simulink model "ctrl_student_HIL"  (R2015a)
settings: Solver=ode3  StartTime=0.0  StopTime=inf  RelTol=1e-3
libraries: dspstat3 x1, simulink x1
(part 2 of 3)

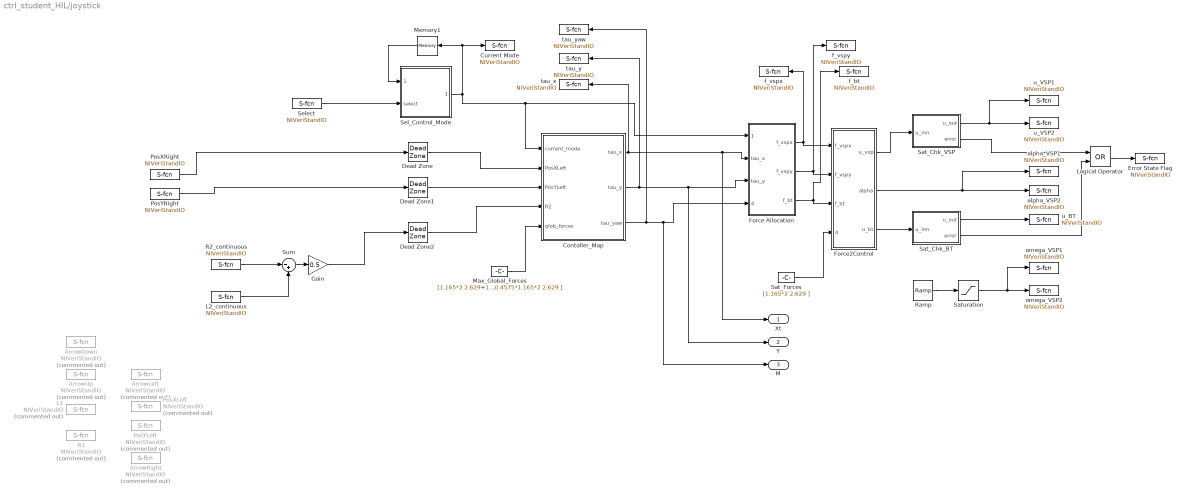
== system ctrl_student_HIL/joystick ==
  ArrowDown : S-Function  Priority=9  Commented=on  FunctionName=NIVeriStandIO  Parameters=width dtype portnum stime stype btype  mask(NI VeriStand Inport){portnum=9, width=-1, stime=-1, dtype=auto, stype=auto, btype=1}
      mask prompts: portnum "Port number:"; width "Port dimensions (-1 for dynamically sized):"; stime "Sample time (-1 for inherited):"; dtype "Data type:"; stype "Signal type:"; btype "Block type:"
      mask help: Use this inport on any level of nested subsystems to allow NI VeriStand software to map signals to it.
      mask init:
      | NIVeriStandIO_init;
      settings: CopyFcn=NIVeriStand_MDL_functions('', 'IO_copy');  DeleteFcn=NIVeriStand_MDL_functions('', 'IO_delete');  MoveFcn=set_param(gcb, 'Mask', 'on');
      mask Callback portnum: NIVeriStand_MDL_functions('', 'IO_setportnum');
      mask TypeOptions dtype: auto | double | single | int8 | uint8 | int16 | uint16 | int32 | uint32 | boolean
      mask Callback dtype: NIVeriStand_MDL_functions('', 'IO_booleansignal');
      mask TypeOptions stype: auto | real | complex
      mask Display:
      | patch([-x x], [-y y], [.90980 .81960 .32156]);
      | plot([xrad -x x xrad], [yrad -y y yrad]);
      | fprintf('NI In%d', portnum);
  ArrowLeft : S-Function  Priority=11  Commented=on  FunctionName=NIVeriStandIO  Parameters=width dtype portnum stime stype btype  mask(NI VeriStand Inport){portnum=11, width=-1, stime=-1, dtype=auto, stype=auto, btype=1}
      mask prompts: portnum "Port number:"; width "Port dimensions (-1 for dynamically sized):"; stime "Sample time (-1 for inherited):"; dtype "Data type:"; stype "Signal type:"; btype "Block type:"
      mask help: Use this inport on any level of nested subsystems to allow NI VeriStand software to map signals to it.
      mask init:
      | NIVeriStandIO_init;
      settings: CopyFcn=NIVeriStand_MDL_functions('', 'IO_copy');  DeleteFcn=NIVeriStand_MDL_functions('', 'IO_delete');  MoveFcn=set_param(gcb, 'Mask', 'on');
      mask Callback portnum: NIVeriStand_MDL_functions('', 'IO_setportnum');
      mask TypeOptions dtype: auto | double | single | int8 | uint8 | int16 | uint16 | int32 | uint32 | boolean
      mask Callback dtype: NIVeriStand_MDL_functions('', 'IO_booleansignal');
      mask TypeOptions stype: auto | real | complex
      mask Display:
      | patch([-x x], [-y y], [.90980 .81960 .32156]);
      | plot([xrad -x x xrad], [yrad -y y yrad]);
      | fprintf('NI In%d', portnum);
  ArrowRight : S-Function  Priority=12  Commented=on  FunctionName=NIVeriStandIO  Parameters=width dtype portnum stime stype btype  mask(NI VeriStand Inport){portnum=12, width=-1, stime=-1, dtype=auto, stype=auto, btype=1}
      mask prompts: portnum "Port number:"; width "Port dimensions (-1 for dynamically sized):"; stime "Sample time (-1 for inherited):"; dtype "Data type:"; stype "Signal type:"; btype "Block type:"
      mask help: Use this inport on any level of nested subsystems to allow NI VeriStand software to map signals to it.
      mask init:
      | NIVeriStandIO_init;
      settings: CopyFcn=NIVeriStand_MDL_functions('', 'IO_copy');  DeleteFcn=NIVeriStand_MDL_functions('', 'IO_delete');  MoveFcn=set_param(gcb, 'Mask', 'on');
      mask Callback portnum: NIVeriStand_MDL_functions('', 'IO_setportnum');
      mask TypeOptions dtype: auto | double | single | int8 | uint8 | int16 | uint16 | int32 | uint32 | boolean
      mask Callback dtype: NIVeriStand_MDL_functions('', 'IO_booleansignal');
      mask TypeOptions stype: auto | real | complex
      mask Display:
      | patch([-x x], [-y y], [.90980 .81960 .32156]);
      | plot([xrad -x x xrad], [yrad -y y yrad]);
      | fprintf('NI In%d', portnum);
  ArrowUp : S-Function  Priority=10  Commented=on  FunctionName=NIVeriStandIO  Parameters=width dtype portnum stime stype btype  mask(NI VeriStand Inport){portnum=10, width=-1, stime=-1, dtype=auto, stype=auto, btype=1}
      mask prompts: portnum "Port number:"; width "Port dimensions (-1 for dynamically sized):"; stime "Sample time (-1 for inherited):"; dtype "Data type:"; stype "Signal type:"; btype "Block type:"
      mask help: Use this inport on any level of nested subsystems to allow NI VeriStand software to map signals to it.
      mask init:
      | NIVeriStandIO_init;
      settings: CopyFcn=NIVeriStand_MDL_functions('', 'IO_copy');  DeleteFcn=NIVeriStand_MDL_functions('', 'IO_delete');  MoveFcn=set_param(gcb, 'Mask', 'on');
      mask Callback portnum: NIVeriStand_MDL_functions('', 'IO_setportnum');
      mask TypeOptions dtype: auto | double | single | int8 | uint8 | int16 | uint16 | int32 | uint32 | boolean
      mask Callback dtype: NIVeriStand_MDL_functions('', 'IO_booleansignal');
      mask TypeOptions stype: auto | real | complex
      mask Display:
      | patch([-x x], [-y y], [.90980 .81960 .32156]);
      | plot([xrad -x x xrad], [yrad -y y yrad]);
      | fprintf('NI In%d', portnum);
  Contoller_Map : MATLAB Function  TreatAsAtomicUnit=on
  "Current Mode " : S-Function  Priority=8  FunctionName=NIVeriStandIO  Parameters=width dtype portnum stime stype btype  mask(NI VeriStand Outport){portnum=8, width=-1, stime=-1, dtype=auto, stype=auto, btype=0}
      mask prompts: portnum "Port number:"; width "Port dimensions (-1 for dynamically sized):"; stime "Sample time (-1 for inherited):"; dtype "Data type:"; stype "Signal type:"; btype "Block type:"
      mask help: Use this outport on any level of nested subsystems to allow NI VeriStand software to map signals to it.
      mask init:
      | NIVeriStandIO_init;
      settings: CopyFcn=NIVeriStand_MDL_functions('', 'IO_copy');  DeleteFcn=NIVeriStand_MDL_functions('', 'IO_delete');  MoveFcn=set_param(gcb, 'Mask', 'on');
      mask Callback portnum: NIVeriStand_MDL_functions('', 'IO_setportnum');
      mask TypeOptions dtype: auto | double | single | int8 | uint8 | int16 | uint16 | int32 | uint32 | boolean
      mask Callback dtype: NIVeriStand_MDL_functions('', 'IO_booleansignal');
      mask TypeOptions stype: auto | real | complex
      mask Display:
      | patch([-x x], [-y y], [.90980 .81960 .32156]);
      | plot([xrad -x x xrad], [yrad -y y yrad]);
      | fprintf('NI Out%d', portnum);
  Dead Zone : DeadZone  LowerValue=-0.05  UpperValue=0.05  SaturateOnIntegerOverflow=on
  Dead Zone1 : DeadZone  LowerValue=-0.05  UpperValue=0.05  SaturateOnIntegerOverflow=on
  Dead Zone2 : DeadZone  LowerValue=-0.05  UpperValue=0.05  SaturateOnIntegerOverflow=on
  Error State Flag : S-Function  Priority=9  FunctionName=NIVeriStandIO  Parameters=width dtype portnum stime stype btype  mask(NI VeriStand Outport){portnum=9, width=-1, stime=-1, dtype=boolean, stype=auto, btype=0}
      mask prompts: portnum "Port number:"; width "Port dimensions (-1 for dynamically sized):"; stime "Sample time (-1 for inherited):"; dtype "Data type:"; stype "Signal type:"; btype "Block type:"
      mask help: Use this outport on any level of nested subsystems to allow NI VeriStand software to map signals to it.
      mask init:
      | NIVeriStandIO_init;
      settings: CopyFcn=NIVeriStand_MDL_functions('', 'IO_copy');  DeleteFcn=NIVeriStand_MDL_functions('', 'IO_delete');  MoveFcn=set_param(gcb, 'Mask', 'on');
      mask Callback portnum: NIVeriStand_MDL_functions('', 'IO_setportnum');
      mask TypeOptions dtype: auto | double | single | int8 | uint8 | int16 | uint16 | int32 | uint32 | boolean
      mask Callback dtype: NIVeriStand_MDL_functions('', 'IO_booleansignal');
      mask TypeOptions stype: auto | real | complex
      mask Display:
      | patch([-x x], [-y y], [.90980 .81960 .32156]);
      | plot([xrad -x x xrad], [yrad -y y yrad]);
      | fprintf('NI Out%d', portnum);
  Force Allocation : MATLAB Function  TreatAsAtomicUnit=on
  Force2Control : MATLAB Function  TreatAsAtomicUnit=on
  Gain : Gain  Gain=0.5
  L1 : S-Function  Priority=7  Commented=on  FunctionName=NIVeriStandIO  Parameters=width dtype portnum stime stype btype  mask(NI VeriStand Inport){portnum=7, width=-1, stime=-1, dtype=auto, stype=auto, btype=1}
      mask prompts: portnum "Port number:"; width "Port dimensions (-1 for dynamically sized):"; stime "Sample time (-1 for inherited):"; dtype "Data type:"; stype "Signal type:"; btype "Block type:"
      mask help: Use this inport on any level of nested subsystems to allow NI VeriStand software to map signals to it.
      mask init:
      | NIVeriStandIO_init;
      settings: CopyFcn=NIVeriStand_MDL_functions('', 'IO_copy');  DeleteFcn=NIVeriStand_MDL_functions('', 'IO_delete');  MoveFcn=set_param(gcb, 'Mask', 'on');
      mask Callback portnum: NIVeriStand_MDL_functions('', 'IO_setportnum');
      mask TypeOptions dtype: auto | double | single | int8 | uint8 | int16 | uint16 | int32 | uint32 | boolean
      mask Callback dtype: NIVeriStand_MDL_functions('', 'IO_booleansignal');
      mask TypeOptions stype: auto | real | complex
      mask Display:
      | patch([-x x], [-y y], [.90980 .81960 .32156]);
      | plot([xrad -x x xrad], [yrad -y y yrad]);
      | fprintf('NI In%d', portnum);
  L2_continuous : S-Function  Priority=1  FunctionName=NIVeriStandIO  Parameters=width dtype portnum stime stype btype  mask(NI VeriStand Inport){portnum=1, width=-1, stime=-1, dtype=auto, stype=auto, btype=1}
      mask prompts: portnum "Port number:"; width "Port dimensions (-1 for dynamically sized):"; stime "Sample time (-1 for inherited):"; dtype "Data type:"; stype "Signal type:"; btype "Block type:"
      mask help: Use this inport on any level of nested subsystems to allow NI VeriStand software to map signals to it.
      mask init:
      | NIVeriStandIO_init;
      settings: CopyFcn=NIVeriStand_MDL_functions('', 'IO_copy');  DeleteFcn=NIVeriStand_MDL_functions('', 'IO_delete');  MoveFcn=set_param(gcb, 'Mask', 'on');
      mask Callback portnum: NIVeriStand_MDL_functions('', 'IO_setportnum');
      mask TypeOptions dtype: auto | double | single | int8 | uint8 | int16 | uint16 | int32 | uint32 | boolean
      mask Callback dtype: NIVeriStand_MDL_functions('', 'IO_booleansignal');
      mask TypeOptions stype: auto | real | complex
      mask Display:
      | patch([-x x], [-y y], [.90980 .81960 .32156]);
      | plot([xrad -x x xrad], [yrad -y y yrad]);
      | fprintf('NI In%d', portnum);
  Logical Operator : Logic  Operator=OR  AllPortsSameDT=off  OutDataTypeStr=boolean
  Max_Global_Forces : Constant  Value=[1.165*2 2.629+1.165*2 0.3875*2.629+0.4575*1.165*2 2.629 ]
  Memory1 : Memory  X0=2
  PosXLeft : S-Function  Priority=5  Commented=on  FunctionName=NIVeriStandIO  Parameters=width dtype portnum stime stype btype  mask(NI VeriStand Inport){portnum=5, width=-1, stime=-1, dtype=auto, stype=auto, btype=1}
      mask prompts: portnum "Port number:"; width "Port dimensions (-1 for dynamically sized):"; stime "Sample time (-1 for inherited):"; dtype "Data type:"; stype "Signal type:"; btype "Block type:"
      mask help: Use this inport on any level of nested subsystems to allow NI VeriStand software to map signals to it.
      mask init:
      | NIVeriStandIO_init;
      settings: CopyFcn=NIVeriStand_MDL_functions('', 'IO_copy');  DeleteFcn=NIVeriStand_MDL_functions('', 'IO_delete');  MoveFcn=set_param(gcb, 'Mask', 'on');
      mask Callback portnum: NIVeriStand_MDL_functions('', 'IO_setportnum');
      mask TypeOptions dtype: auto | double | single | int8 | uint8 | int16 | uint16 | int32 | uint32 | boolean
      mask Callback dtype: NIVeriStand_MDL_functions('', 'IO_booleansignal');
      mask TypeOptions stype: auto | real | complex
      mask Display:
      | patch([-x x], [-y y], [.90980 .81960 .32156]);
      | plot([xrad -x x xrad], [yrad -y y yrad]);
      | fprintf('NI In%d', portnum);
  PosXRight : S-Function  Priority=2  FunctionName=NIVeriStandIO  Parameters=width dtype portnum stime stype btype  mask(NI VeriStand Inport){portnum=2, width=-1, stime=-1, dtype=auto, stype=auto, btype=1}
      mask prompts: portnum "Port number:"; width "Port dimensions (-1 for dynamically sized):"; stime "Sample time (-1 for inherited):"; dtype "Data type:"; stype "Signal type:"; btype "Block type:"
      mask help: Use this inport on any level of nested subsystems to allow NI VeriStand software to map signals to it.
      mask init:
      | NIVeriStandIO_init;
      settings: CopyFcn=NIVeriStand_MDL_functions('', 'IO_copy');  DeleteFcn=NIVeriStand_MDL_functions('', 'IO_delete');  MoveFcn=set_param(gcb, 'Mask', 'on');
      mask Callback portnum: NIVeriStand_MDL_functions('', 'IO_setportnum');
      mask TypeOptions dtype: auto | double | single | int8 | uint8 | int16 | uint16 | int32 | uint32 | boolean
      mask Callback dtype: NIVeriStand_MDL_functions('', 'IO_booleansignal');
      mask TypeOptions stype: auto | real | complex
      mask Display:
      | patch([-x x], [-y y], [.90980 .81960 .32156]);
      | plot([xrad -x x xrad], [yrad -y y yrad]);
      | fprintf('NI In%d', portnum);
  PosYLeft : S-Function  Priority=6  Commented=on  FunctionName=NIVeriStandIO  Parameters=width dtype portnum stime stype btype  mask(NI VeriStand Inport){portnum=6, width=-1, stime=-1, dtype=auto, stype=auto, btype=1}
      mask prompts: portnum "Port number:"; width "Port dimensions (-1 for dynamically sized):"; stime "Sample time (-1 for inherited):"; dtype "Data type:"; stype "Signal type:"; btype "Block type:"
      mask help: Use this inport on any level of nested subsystems to allow NI VeriStand software to map signals to it.
      mask init:
      | NIVeriStandIO_init;
      settings: CopyFcn=NIVeriStand_MDL_functions('', 'IO_copy');  DeleteFcn=NIVeriStand_MDL_functions('', 'IO_delete');  MoveFcn=set_param(gcb, 'Mask', 'on');
      mask Callback portnum: NIVeriStand_MDL_functions('', 'IO_setportnum');
      mask TypeOptions dtype: auto | double | single | int8 | uint8 | int16 | uint16 | int32 | uint32 | boolean
      mask Callback dtype: NIVeriStand_MDL_functions('', 'IO_booleansignal');
      mask TypeOptions stype: auto | real | complex
      mask Display:
      | patch([-x x], [-y y], [.90980 .81960 .32156]);
      | plot([xrad -x x xrad], [yrad -y y yrad]);
      | fprintf('NI In%d', portnum);
  PosYRight : S-Function  Priority=3  FunctionName=NIVeriStandIO  Parameters=width dtype portnum stime stype btype  mask(NI VeriStand Inport){portnum=3, width=-1, stime=-1, dtype=auto, stype=auto, btype=1}
      mask prompts: portnum "Port number:"; width "Port dimensions (-1 for dynamically sized):"; stime "Sample time (-1 for inherited):"; dtype "Data type:"; stype "Signal type:"; btype "Block type:"
      mask help: Use this inport on any level of nested subsystems to allow NI VeriStand software to map signals to it.
      mask init:
      | NIVeriStandIO_init;
      settings: CopyFcn=NIVeriStand_MDL_functions('', 'IO_copy');  DeleteFcn=NIVeriStand_MDL_functions('', 'IO_delete');  MoveFcn=set_param(gcb, 'Mask', 'on');
      mask Callback portnum: NIVeriStand_MDL_functions('', 'IO_setportnum');
      mask TypeOptions dtype: auto | double | single | int8 | uint8 | int16 | uint16 | int32 | uint32 | boolean
      mask Callback dtype: NIVeriStand_MDL_functions('', 'IO_booleansignal');
      mask TypeOptions stype: auto | real | complex
      mask Display:
      | patch([-x x], [-y y], [.90980 .81960 .32156]);
      | plot([xrad -x x xrad], [yrad -y y yrad]);
      | fprintf('NI In%d', portnum);
  R1 : S-Function  Priority=8  Commented=on  FunctionName=NIVeriStandIO  Parameters=width dtype portnum stime stype btype  mask(NI VeriStand Inport){portnum=8, width=-1, stime=-1, dtype=auto, stype=auto, btype=1}
      mask prompts: portnum "Port number:"; width "Port dimensions (-1 for dynamically sized):"; stime "Sample time (-1 for inherited):"; dtype "Data type:"; stype "Signal type:"; btype "Block type:"
      mask help: Use this inport on any level of nested subsystems to allow NI VeriStand software to map signals to it.
      mask init:
      | NIVeriStandIO_init;
      settings: CopyFcn=NIVeriStand_MDL_functions('', 'IO_copy');  DeleteFcn=NIVeriStand_MDL_functions('', 'IO_delete');  MoveFcn=set_param(gcb, 'Mask', 'on');
      mask Callback portnum: NIVeriStand_MDL_functions('', 'IO_setportnum');
      mask TypeOptions dtype: auto | double | single | int8 | uint8 | int16 | uint16 | int32 | uint32 | boolean
      mask Callback dtype: NIVeriStand_MDL_functions('', 'IO_booleansignal');
      mask TypeOptions stype: auto | real | complex
      mask Display:
      | patch([-x x], [-y y], [.90980 .81960 .32156]);
      | plot([xrad -x x xrad], [yrad -y y yrad]);
      | fprintf('NI In%d', portnum);
  R2_continuous : S-Function  Priority=4  FunctionName=NIVeriStandIO  Parameters=width dtype portnum stime stype btype  mask(NI VeriStand Inport){portnum=4, width=-1, stime=-1, dtype=auto, stype=auto, btype=1}
      mask prompts: portnum "Port number:"; width "Port dimensions (-1 for dynamically sized):"; stime "Sample time (-1 for inherited):"; dtype "Data type:"; stype "Signal type:"; btype "Block type:"
      mask help: Use this inport on any level of nested subsystems to allow NI VeriStand software to map signals to it.
      mask init:
      | NIVeriStandIO_init;
      settings: CopyFcn=NIVeriStand_MDL_functions('', 'IO_copy');  DeleteFcn=NIVeriStand_MDL_functions('', 'IO_delete');  MoveFcn=set_param(gcb, 'Mask', 'on');
      mask Callback portnum: NIVeriStand_MDL_functions('', 'IO_setportnum');
      mask TypeOptions dtype: auto | double | single | int8 | uint8 | int16 | uint16 | int32 | uint32 | boolean
      mask Callback dtype: NIVeriStand_MDL_functions('', 'IO_booleansignal');
      mask TypeOptions stype: auto | real | complex
      mask Display:
      | patch([-x x], [-y y], [.90980 .81960 .32156]);
      | plot([xrad -x x xrad], [yrad -y y yrad]);
      | fprintf('NI In%d', portnum);
  Ramp : simulink/Sources/Ramp  slope=0.1  start=0  X0=0
  Sat_Chk_BT : MATLAB Function  TreatAsAtomicUnit=on
  Sat_Chk_VSP : MATLAB Function  TreatAsAtomicUnit=on
  Sat_Forces : Constant  Value=[1.165*2 2.629 ]
  Saturation : Saturate  UpperLimit=0.3  LowerLimit=0
  Sel_Control_Mode : MATLAB Function  TreatAsAtomicUnit=on
  Select : S-Function  Priority=13  FunctionName=NIVeriStandIO  Parameters=width dtype portnum stime stype btype  mask(NI VeriStand Inport){portnum=13, width=-1, stime=-1, dtype=auto, stype=auto, btype=1}
      mask prompts: portnum "Port number:"; width "Port dimensions (-1 for dynamically sized):"; stime "Sample time (-1 for inherited):"; dtype "Data type:"; stype "Signal type:"; btype "Block type:"
      mask help: Use this inport on any level of nested subsystems to allow NI VeriStand software to map signals to it.
      mask init:
      | NIVeriStandIO_init;
      settings: CopyFcn=NIVeriStand_MDL_functions('', 'IO_copy');  DeleteFcn=NIVeriStand_MDL_functions('', 'IO_delete');  MoveFcn=set_param(gcb, 'Mask', 'on');
      mask Callback portnum: NIVeriStand_MDL_functions('', 'IO_setportnum');
      mask TypeOptions dtype: auto | double | single | int8 | uint8 | int16 | uint16 | int32 | uint32 | boolean
      mask Callback dtype: NIVeriStand_MDL_functions('', 'IO_booleansignal');
      mask TypeOptions stype: auto | real | complex
      mask Display:
      | patch([-x x], [-y y], [.90980 .81960 .32156]);
      | plot([xrad -x x xrad], [yrad -y y yrad]);
      | fprintf('NI In%d', portnum);
  Sum : Sum  Inputs=|-+
  alpha_VSP1 : S-Function  Priority=4  FunctionName=NIVeriStandIO  Parameters=width dtype portnum stime stype btype  mask(NI VeriStand Outport){portnum=4, width=-1, stime=-1, dtype=auto, stype=auto, btype=0}
      mask prompts: portnum "Port number:"; width "Port dimensions (-1 for dynamically sized):"; stime "Sample time (-1 for inherited):"; dtype "Data type:"; stype "Signal type:"; btype "Block type:"
      mask help: Use this outport on any level of nested subsystems to allow NI VeriStand software to map signals to it.
      mask init:
      | NIVeriStandIO_init;
      settings: CopyFcn=NIVeriStand_MDL_functions('', 'IO_copy');  DeleteFcn=NIVeriStand_MDL_functions('', 'IO_delete');  MoveFcn=set_param(gcb, 'Mask', 'on');
      mask Callback portnum: NIVeriStand_MDL_functions('', 'IO_setportnum');
      mask TypeOptions dtype: auto | double | single | int8 | uint8 | int16 | uint16 | int32 | uint32 | boolean
      mask Callback dtype: NIVeriStand_MDL_functions('', 'IO_booleansignal');
      mask TypeOptions stype: auto | real | complex
      mask Display:
      | patch([-x x], [-y y], [.90980 .81960 .32156]);
      | plot([xrad -x x xrad], [yrad -y y yrad]);
      | fprintf('NI Out%d', portnum);
  alpha_VSP2 : S-Function  Priority=5  FunctionName=NIVeriStandIO  Parameters=width dtype portnum stime stype btype  mask(NI VeriStand Outport){portnum=5, width=-1, stime=-1, dtype=auto, stype=auto, btype=0}
      mask prompts: portnum "Port number:"; width "Port dimensions (-1 for dynamically sized):"; stime "Sample time (-1 for inherited):"; dtype "Data type:"; stype "Signal type:"; btype "Block type:"
      mask help: Use this outport on any level of nested subsystems to allow NI VeriStand software to map signals to it.
      mask init:
      | NIVeriStandIO_init;
      settings: CopyFcn=NIVeriStand_MDL_functions('', 'IO_copy');  DeleteFcn=NIVeriStand_MDL_functions('', 'IO_delete');  MoveFcn=set_param(gcb, 'Mask', 'on');
      mask Callback portnum: NIVeriStand_MDL_functions('', 'IO_setportnum');
      mask TypeOptions dtype: auto | double | single | int8 | uint8 | int16 | uint16 | int32 | uint32 | boolean
      mask Callback dtype: NIVeriStand_MDL_functions('', 'IO_booleansignal');
      mask TypeOptions stype: auto | real | complex
      mask Display:
      | patch([-x x], [-y y], [.90980 .81960 .32156]);
      | plot([xrad -x x xrad], [yrad -y y yrad]);
      | fprintf('NI Out%d', portnum);
  f_bt : S-Function  Priority=12  FunctionName=NIVeriStandIO  Parameters=width dtype portnum stime stype btype  mask(NI VeriStand Outport){portnum=12, width=-1, stime=-1, dtype=auto, stype=auto, btype=0}
      mask prompts: portnum "Port number:"; width "Port dimensions (-1 for dynamically sized):"; stime "Sample time (-1 for inherited):"; dtype "Data type:"; stype "Signal type:"; btype "Block type:"
      mask help: Use this outport on any level of nested subsystems to allow NI VeriStand software to map signals to it.
      mask init:
      | NIVeriStandIO_init;
      settings: CopyFcn=NIVeriStand_MDL_functions('', 'IO_copy');  DeleteFcn=NIVeriStand_MDL_functions('', 'IO_delete');  MoveFcn=set_param(gcb, 'Mask', 'on');
      mask Callback portnum: NIVeriStand_MDL_functions('', 'IO_setportnum');
      mask TypeOptions dtype: auto | double | single | int8 | uint8 | int16 | uint16 | int32 | uint32 | boolean
      mask Callback dtype: NIVeriStand_MDL_functions('', 'IO_booleansignal');
      mask TypeOptions stype: auto | real | complex
      mask Display:
      | patch([-x x], [-y y], [.90980 .81960 .32156]);
      | plot([xrad -x x xrad], [yrad -y y yrad]);
      | fprintf('NI Out%d', portnum);
  f_vspx : S-Function  Priority=10  FunctionName=NIVeriStandIO  Parameters=width dtype portnum stime stype btype  mask(NI VeriStand Outport){portnum=10, width=-1, stime=-1, dtype=auto, stype=auto, btype=0}
      mask prompts: portnum "Port number:"; width "Port dimensions (-1 for dynamically sized):"; stime "Sample time (-1 for inherited):"; dtype "Data type:"; stype "Signal type:"; btype "Block type:"
      mask help: Use this outport on any level of nested subsystems to allow NI VeriStand software to map signals to it.
      mask init:
      | NIVeriStandIO_init;
      settings: CopyFcn=NIVeriStand_MDL_functions('', 'IO_copy');  DeleteFcn=NIVeriStand_MDL_functions('', 'IO_delete');  MoveFcn=set_param(gcb, 'Mask', 'on');
      mask Callback portnum: NIVeriStand_MDL_functions('', 'IO_setportnum');
      mask TypeOptions dtype: auto | double | single | int8 | uint8 | int16 | uint16 | int32 | uint32 | boolean
      mask Callback dtype: NIVeriStand_MDL_functions('', 'IO_booleansignal');
      mask TypeOptions stype: auto | real | complex
      mask Display:
      | patch([-x x], [-y y], [.90980 .81960 .32156]);
      | plot([xrad -x x xrad], [yrad -y y yrad]);
      | fprintf('NI Out%d', portnum);
  f_vspy : S-Function  Priority=11  FunctionName=NIVeriStandIO  Parameters=width dtype portnum stime stype btype  mask(NI VeriStand Outport){portnum=11, width=-1, stime=-1, dtype=auto, stype=auto, btype=0}
      mask prompts: portnum "Port number:"; width "Port dimensions (-1 for dynamically sized):"; stime "Sample time (-1 for inherited):"; dtype "Data type:"; stype "Signal type:"; btype "Block type:"
      mask help: Use this outport on any level of nested subsystems to allow NI VeriStand software to map signals to it.
      mask init:
      | NIVeriStandIO_init;
      settings: CopyFcn=NIVeriStand_MDL_functions('', 'IO_copy');  DeleteFcn=NIVeriStand_MDL_functions('', 'IO_delete');  MoveFcn=set_param(gcb, 'Mask', 'on');
      mask Callback portnum: NIVeriStand_MDL_functions('', 'IO_setportnum');
      mask TypeOptions dtype: auto | double | single | int8 | uint8 | int16 | uint16 | int32 | uint32 | boolean
      mask Callback dtype: NIVeriStand_MDL_functions('', 'IO_booleansignal');
      mask TypeOptions stype: auto | real | complex
      mask Display:
      | patch([-x x], [-y y], [.90980 .81960 .32156]);
      | plot([xrad -x x xrad], [yrad -y y yrad]);
      | fprintf('NI Out%d', portnum);
  omega_VSP1 : S-Function  Priority=6  FunctionName=NIVeriStandIO  Parameters=width dtype portnum stime stype btype  mask(NI VeriStand Outport){portnum=6, width=-1, stime=-1, dtype=auto, stype=auto, btype=0}
      mask prompts: portnum "Port number:"; width "Port dimensions (-1 for dynamically sized):"; stime "Sample time (-1 for inherited):"; dtype "Data type:"; stype "Signal type:"; btype "Block type:"
      mask help: Use this outport on any level of nested subsystems to allow NI VeriStand software to map signals to it.
      mask init:
      | NIVeriStandIO_init;
      settings: CopyFcn=NIVeriStand_MDL_functions('', 'IO_copy');  DeleteFcn=NIVeriStand_MDL_functions('', 'IO_delete');  MoveFcn=set_param(gcb, 'Mask', 'on');
      mask Callback portnum: NIVeriStand_MDL_functions('', 'IO_setportnum');
      mask TypeOptions dtype: auto | double | single | int8 | uint8 | int16 | uint16 | int32 | uint32 | boolean
      mask Callback dtype: NIVeriStand_MDL_functions('', 'IO_booleansignal');
      mask TypeOptions stype: auto | real | complex
      mask Display:
      | patch([-x x], [-y y], [.90980 .81960 .32156]);
      | plot([xrad -x x xrad], [yrad -y y yrad]);
      | fprintf('NI Out%d', portnum);
  omega_VSP2 : S-Function  Priority=7  FunctionName=NIVeriStandIO  Parameters=width dtype portnum stime stype btype  mask(NI VeriStand Outport){portnum=7, width=-1, stime=-1, dtype=auto, stype=auto, btype=0}
      mask prompts: portnum "Port number:"; width "Port dimensions (-1 for dynamically sized):"; stime "Sample time (-1 for inherited):"; dtype "Data type:"; stype "Signal type:"; btype "Block type:"
      mask help: Use this outport on any level of nested subsystems to allow NI VeriStand software to map signals to it.
      mask init:
      | NIVeriStandIO_init;
      settings: CopyFcn=NIVeriStand_MDL_functions('', 'IO_copy');  DeleteFcn=NIVeriStand_MDL_functions('', 'IO_delete');  MoveFcn=set_param(gcb, 'Mask', 'on');
      mask Callback portnum: NIVeriStand_MDL_functions('', 'IO_setportnum');
      mask TypeOptions dtype: auto | double | single | int8 | uint8 | int16 | uint16 | int32 | uint32 | boolean
      mask Callback dtype: NIVeriStand_MDL_functions('', 'IO_booleansignal');
      mask TypeOptions stype: auto | real | complex
      mask Display:
      | patch([-x x], [-y y], [.90980 .81960 .32156]);
      | plot([xrad -x x xrad], [yrad -y y yrad]);
      | fprintf('NI Out%d', portnum);
  tau_x : S-Function  Priority=14  FunctionName=NIVeriStandIO  Parameters=width dtype portnum stime stype btype  mask(NI VeriStand Outport){portnum=14, width=-1, stime=-1, dtype=auto, stype=auto, btype=0}
      mask prompts: portnum "Port number:"; width "Port dimensions (-1 for dynamically sized):"; stime "Sample time (-1 for inherited):"; dtype "Data type:"; stype "Signal type:"; btype "Block type:"
      mask help: Use this outport on any level of nested subsystems to allow NI VeriStand software to map signals to it.
      mask init:
      | NIVeriStandIO_init;
      settings: CopyFcn=NIVeriStand_MDL_functions('', 'IO_copy');  DeleteFcn=NIVeriStand_MDL_functions('', 'IO_delete');  MoveFcn=set_param(gcb, 'Mask', 'on');
      mask Callback portnum: NIVeriStand_MDL_functions('', 'IO_setportnum');
      mask TypeOptions dtype: auto | double | single | int8 | uint8 | int16 | uint16 | int32 | uint32 | boolean
      mask Callback dtype: NIVeriStand_MDL_functions('', 'IO_booleansignal');
      mask TypeOptions stype: auto | real | complex
      mask Display:
      | patch([-x x], [-y y], [.90980 .81960 .32156]);
      | plot([xrad -x x xrad], [yrad -y y yrad]);
      | fprintf('NI Out%d', portnum);
  tau_y : S-Function  Priority=15  FunctionName=NIVeriStandIO  Parameters=width dtype portnum stime stype btype  mask(NI VeriStand Outport){portnum=15, width=-1, stime=-1, dtype=auto, stype=auto, btype=0}
      mask prompts: portnum "Port number:"; width "Port dimensions (-1 for dynamically sized):"; stime "Sample time (-1 for inherited):"; dtype "Data type:"; stype "Signal type:"; btype "Block type:"
      mask help: Use this outport on any level of nested subsystems to allow NI VeriStand software to map signals to it.
      mask init:
      | NIVeriStandIO_init;
      settings: CopyFcn=NIVeriStand_MDL_functions('', 'IO_copy');  DeleteFcn=NIVeriStand_MDL_functions('', 'IO_delete');  MoveFcn=set_param(gcb, 'Mask', 'on');
      mask Callback portnum: NIVeriStand_MDL_functions('', 'IO_setportnum');
      mask TypeOptions dtype: auto | double | single | int8 | uint8 | int16 | uint16 | int32 | uint32 | boolean
      mask Callback dtype: NIVeriStand_MDL_functions('', 'IO_booleansignal');
      mask TypeOptions stype: auto | real | complex
      mask Display:
      | patch([-x x], [-y y], [.90980 .81960 .32156]);
      | plot([xrad -x x xrad], [yrad -y y yrad]);
      | fprintf('NI Out%d', portnum);
  tau_yaw : S-Function  Priority=13  FunctionName=NIVeriStandIO  Parameters=width dtype portnum stime stype btype  mask(NI VeriStand Outport){portnum=13, width=-1, stime=-1, dtype=auto, stype=auto, btype=0}
      mask prompts: portnum "Port number:"; width "Port dimensions (-1 for dynamically sized):"; stime "Sample time (-1 for inherited):"; dtype "Data type:"; stype "Signal type:"; btype "Block type:"
      mask help: Use this outport on any level of nested subsystems to allow NI VeriStand software to map signals to it.
      mask init:
      | NIVeriStandIO_init;
      settings: CopyFcn=NIVeriStand_MDL_functions('', 'IO_copy');  DeleteFcn=NIVeriStand_MDL_functions('', 'IO_delete');  MoveFcn=set_param(gcb, 'Mask', 'on');
      mask Callback portnum: NIVeriStand_MDL_functions('', 'IO_setportnum');
      mask TypeOptions dtype: auto | double | single | int8 | uint8 | int16 | uint16 | int32 | uint32 | boolean
      mask Callback dtype: NIVeriStand_MDL_functions('', 'IO_booleansignal');
      mask TypeOptions stype: auto | real | complex
      mask Display:
      | patch([-x x], [-y y], [.90980 .81960 .32156]);
      | plot([xrad -x x xrad], [yrad -y y yrad]);
      | fprintf('NI Out%d', portnum);
  u_BT : S-Function  Priority=1  FunctionName=NIVeriStandIO  Parameters=width dtype portnum stime stype btype  mask(NI VeriStand Outport){portnum=1, width=-1, stime=-1, dtype=auto, stype=auto, btype=0}
      mask prompts: portnum "Port number:"; width "Port dimensions (-1 for dynamically sized):"; stime "Sample time (-1 for inherited):"; dtype "Data type:"; stype "Signal type:"; btype "Block type:"
      mask help: Use this outport on any level of nested subsystems to allow NI VeriStand software to map signals to it.
      mask init:
      | NIVeriStandIO_init;
      settings: CopyFcn=NIVeriStand_MDL_functions('', 'IO_copy');  DeleteFcn=NIVeriStand_MDL_functions('', 'IO_delete');  MoveFcn=set_param(gcb, 'Mask', 'on');
      mask Callback portnum: NIVeriStand_MDL_functions('', 'IO_setportnum');
      mask TypeOptions dtype: auto | double | single | int8 | uint8 | int16 | uint16 | int32 | uint32 | boolean
      mask Callback dtype: NIVeriStand_MDL_functions('', 'IO_booleansignal');
      mask TypeOptions stype: auto | real | complex
      mask Display:
      | patch([-x x], [-y y], [.90980 .81960 .32156]);
      | plot([xrad -x x xrad], [yrad -y y yrad]);
      | fprintf('NI Out%d', portnum);
  u_VSP1 : S-Function  Priority=2  FunctionName=NIVeriStandIO  Parameters=width dtype portnum stime stype btype  mask(NI VeriStand Outport){portnum=2, width=-1, stime=-1, dtype=auto, stype=auto, btype=0}
      mask prompts: portnum "Port number:"; width "Port dimensions (-1 for dynamically sized):"; stime "Sample time (-1 for inherited):"; dtype "Data type:"; stype "Signal type:"; btype "Block type:"
      mask help: Use this outport on any level of nested subsystems to allow NI VeriStand software to map signals to it.
      mask init:
      | NIVeriStandIO_init;
      settings: CopyFcn=NIVeriStand_MDL_functions('', 'IO_copy');  DeleteFcn=NIVeriStand_MDL_functions('', 'IO_delete');  MoveFcn=set_param(gcb, 'Mask', 'on');
      mask Callback portnum: NIVeriStand_MDL_functions('', 'IO_setportnum');
      mask TypeOptions dtype: auto | double | single | int8 | uint8 | int16 | uint16 | int32 | uint32 | boolean
      mask Callback dtype: NIVeriStand_MDL_functions('', 'IO_booleansignal');
      mask TypeOptions stype: auto | real | complex
      mask Display:
      | patch([-x x], [-y y], [.90980 .81960 .32156]);
      | plot([xrad -x x xrad], [yrad -y y yrad]);
      | fprintf('NI Out%d', portnum);
  u_VSP2 : S-Function  Priority=3  FunctionName=NIVeriStandIO  Parameters=width dtype portnum stime stype btype  mask(NI VeriStand Outport){portnum=3, width=-1, stime=-1, dtype=auto, stype=auto, btype=0}
      mask prompts: portnum "Port number:"; width "Port dimensions (-1 for dynamically sized):"; stime "Sample time (-1 for inherited):"; dtype "Data type:"; stype "Signal type:"; btype "Block type:"
      mask help: Use this outport on any level of nested subsystems to allow NI VeriStand software to map signals to it.
      mask init:
      | NIVeriStandIO_init;
      settings: CopyFcn=NIVeriStand_MDL_functions('', 'IO_copy');  DeleteFcn=NIVeriStand_MDL_functions('', 'IO_delete');  MoveFcn=set_param(gcb, 'Mask', 'on');
      mask Callback portnum: NIVeriStand_MDL_functions('', 'IO_setportnum');
      mask TypeOptions dtype: auto | double | single | int8 | uint8 | int16 | uint16 | int32 | uint32 | boolean
      mask Callback dtype: NIVeriStand_MDL_functions('', 'IO_booleansignal');
      mask TypeOptions stype: auto | real | complex
      mask Display:
      | patch([-x x], [-y y], [.90980 .81960 .32156]);
      | plot([xrad -x x xrad], [yrad -y y yrad]);
      | fprintf('NI Out%d', portnum);
  Xt : Outport
  Y : Outport  Port=2
  M : Outport  Port=3
  wires:
  Force Allocation/1(f_vspx) -> Force2Control/1(f_vspx), f_vspx/1
  Force Allocation/2(f_vspy) -> Force2Control/2(f_vspy), f_vspy/1
  Force Allocation/3(f_bt) -> Force2Control/3(f_bt), f_bt/1
  Force2Control/1(u_vsp) -> Sat_Chk_VSP/1(u_inn)
  Force2Control/3(u_bt) -> Sat_Chk_BT/1(u_inn)
  Force2Control/2(alpha) -> alpha_VSP1/1, alpha_VSP2/1
  Ramp/1 -> Saturation/1
  Saturation/1 -> omega_VSP2/1, omega_VSP1/1
  Sat_Chk_VSP/1(u_out) -> u_VSP1/1, u_VSP2/1
  Sat_Chk_BT/1(u_out) -> u_BT/1
  PosXRight/1 -> Dead Zone/1
  PosYRight/1 -> Dead Zone1/1
  Sat_Forces/1 -> Force2Control/4(sat_forces)
  Dead Zone/1 -> Contoller_Map/2(PosXLeft)
  Dead Zone1/1 -> Contoller_Map/3(PosYLeft)
  Sat_Chk_BT/2(error) -> Logical Operator/2
  Sat_Chk_VSP/2(error) -> Logical Operator/1
  Logical Operator/1 -> Error State Flag/1
  Memory1/1 -> Sel_Control_Mode/1(previous_condition)
  Select/1 -> Sel_Control_Mode/2(select)
  Sel_Control_Mode/1(current_mode) -> Force Allocation/1(current_mode), Contoller_Map/1(current_mode), "Current Mode "/1, Memory1/1
  Dead Zone2/1 -> Contoller_Map/4(R2)
  Max_Global_Forces/1 -> Contoller_Map/5(glob_forces)
  Contoller_Map/1(tau_x) -> tau_x/1, Xt/1, Force Allocation/2(tau_x)
  Contoller_Map/2(tau_y) -> Y/1, Force Allocation/3(tau_y), tau_y/1
  Contoller_Map/3(tau_yaw) -> tau_yaw/1, M/1, Force Allocation/4(tau_yaw)
  L2_continuous/1 -> Sum/2
  Sum/1 -> Gain/1
  R2_continuous/1 -> Sum/1
  Gain/1 -> Dead Zone2/1

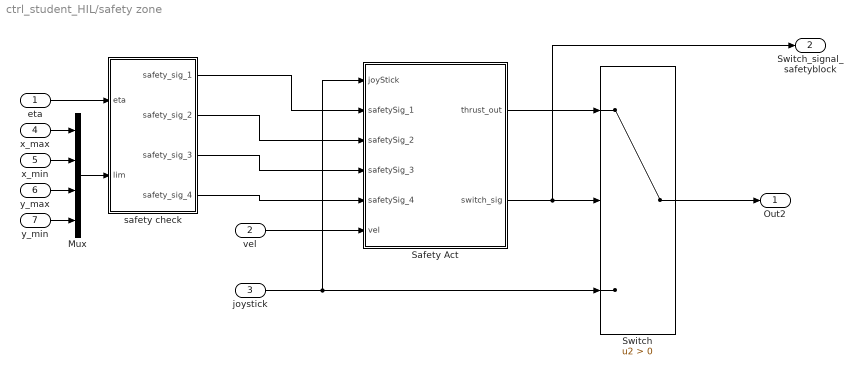
== system ctrl_student_HIL/safety zone  ==
  eta : Inport
  "vel " : Inport  Port=2
  joystick : Inport  Port=3
  x_max : Inport  Port=4
  x_min : Inport  Port=5
  y_max : Inport  Port=6
  y_min : Inport  Port=7
  Mux : Mux
  Safety Act : MATLAB Function  TreatAsAtomicUnit=on
  Switch : Switch  Criteria=u2 > Threshold
  safety check : MATLAB Function  TreatAsAtomicUnit=on
  Out2 : Outport
  Switch_signal_safetyblock : Outport  Port=2
  wires:
  Switch/1 -> Out2/1
  joystick/1 -> Safety Act/1(joyStick), Switch/3
  safety check/1(safety_sig_1) -> Safety Act/2(safetySig_1)
  Safety Act/1(thrust_out) -> Switch/1
  Safety Act/2(switch_sig) -> Switch_signal_safetyblock/1, Switch/2
  safety check/2(safety_sig_2) -> Safety Act/3(safetySig_2)
  safety check/3(safety_sig_3) -> Safety Act/4(safetySig_3)
  safety check/4(safety_sig_4) -> Safety Act/5(safetySig_4)
  "vel "/1 -> Safety Act/6(vel)
  eta/1 -> safety check/1(eta)
  Mux/1 -> safety check/2(lim)
  x_max/1 -> Mux/1
  x_min/1 -> Mux/2
  y_max/1 -> Mux/3
  y_min/1 -> Mux/4

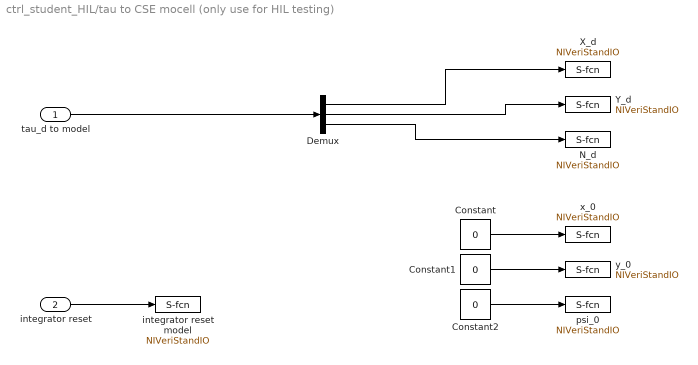
== system ctrl_student_HIL/tau to CSE mocell (only use for HIL testing) ==
  tau_d to model : Inport
  integrator reset : Inport  Port=2
  Constant : Constant  Value=0
  Constant1 : Constant  Value=0
  Constant2 : Constant  Value=0
  Demux : Demux  Outputs=3
  N_d : S-Function  Priority=2  FunctionName=NIVeriStandIO  Parameters=width dtype portnum stime stype btype  mask(NI VeriStand Outport){portnum=2, width=-1, stime=-1, dtype=auto, stype=auto, btype=0}
      mask prompts: portnum "Port number:"; width "Port dimensions (-1 for dynamically sized):"; stime "Sample time (-1 for inherited):"; dtype "Data type:"; stype "Signal type:"; btype "Block type:"
      mask help: Use this outport on any level of nested subsystems to allow NI VeriStand software to map signals to it.
      mask init:
      | NIVeriStandIO_init;
      settings: CopyFcn=NIVeriStand_MDL_functions('', 'IO_copy');  DeleteFcn=NIVeriStand_MDL_functions('', 'IO_delete');  MoveFcn=set_param(gcb, 'Mask', 'on');
      mask Callback portnum: NIVeriStand_MDL_functions('', 'IO_setportnum');
      mask TypeOptions dtype: auto | double | single | int8 | uint8 | int16 | uint16 | int32 | uint32 | boolean
      mask Callback dtype: NIVeriStand_MDL_functions('', 'IO_booleansignal');
      mask TypeOptions stype: auto | real | complex
      mask Display:
      | patch([-x x], [-y y], [.90980 .81960 .32156]);
      | plot([xrad -x x xrad], [yrad -y y yrad]);
      | fprintf('NI Out%d', portnum);
  X_d : S-Function  Priority=1  FunctionName=NIVeriStandIO  Parameters=width dtype portnum stime stype btype  mask(NI VeriStand Outport){portnum=1, width=-1, stime=-1, dtype=auto, stype=auto, btype=0}
      mask prompts: portnum "Port number:"; width "Port dimensions (-1 for dynamically sized):"; stime "Sample time (-1 for inherited):"; dtype "Data type:"; stype "Signal type:"; btype "Block type:"
      mask help: Use this outport on any level of nested subsystems to allow NI VeriStand software to map signals to it.
      mask init:
      | NIVeriStandIO_init;
      settings: CopyFcn=NIVeriStand_MDL_functions('', 'IO_copy');  DeleteFcn=NIVeriStand_MDL_functions('', 'IO_delete');  MoveFcn=set_param(gcb, 'Mask', 'on');
      mask Callback portnum: NIVeriStand_MDL_functions('', 'IO_setportnum');
      mask TypeOptions dtype: auto | double | single | int8 | uint8 | int16 | uint16 | int32 | uint32 | boolean
      mask Callback dtype: NIVeriStand_MDL_functions('', 'IO_booleansignal');
      mask TypeOptions stype: auto | real | complex
      mask Display:
      | patch([-x x], [-y y], [.90980 .81960 .32156]);
      | plot([xrad -x x xrad], [yrad -y y yrad]);
      | fprintf('NI Out%d', portnum);
  Y_d : S-Function  Priority=3  FunctionName=NIVeriStandIO  Parameters=width dtype portnum stime stype btype  mask(NI VeriStand Outport){portnum=3, width=-1, stime=-1, dtype=auto, stype=auto, btype=0}
      mask prompts: portnum "Port number:"; width "Port dimensions (-1 for dynamically sized):"; stime "Sample time (-1 for inherited):"; dtype "Data type:"; stype "Signal type:"; btype "Block type:"
      mask help: Use this outport on any level of nested subsystems to allow NI VeriStand software to map signals to it.
      mask init:
      | NIVeriStandIO_init;
      settings: CopyFcn=NIVeriStand_MDL_functions('', 'IO_copy');  DeleteFcn=NIVeriStand_MDL_functions('', 'IO_delete');  MoveFcn=set_param(gcb, 'Mask', 'on');
      mask Callback portnum: NIVeriStand_MDL_functions('', 'IO_setportnum');
      mask TypeOptions dtype: auto | double | single | int8 | uint8 | int16 | uint16 | int32 | uint32 | boolean
      mask Callback dtype: NIVeriStand_MDL_functions('', 'IO_booleansignal');
      mask TypeOptions stype: auto | real | complex
      mask Display:
      | patch([-x x], [-y y], [.90980 .81960 .32156]);
      | plot([xrad -x x xrad], [yrad -y y yrad]);
      | fprintf('NI Out%d', portnum);
  integrator reset model : S-Function  Priority=7  FunctionName=NIVeriStandIO  Parameters=width dtype portnum stime stype btype  mask(NI VeriStand Outport){portnum=7, width=-1, stime=-1, dtype=auto, stype=auto, btype=0}
      mask prompts: portnum "Port number:"; width "Port dimensions (-1 for dynamically sized):"; stime "Sample time (-1 for inherited):"; dtype "Data type:"; stype "Signal type:"; btype "Block type:"
      mask help: Use this outport on any level of nested subsystems to allow NI VeriStand software to map signals to it.
      mask init:
      | NIVeriStandIO_init;
      settings: CopyFcn=NIVeriStand_MDL_functions('', 'IO_copy');  DeleteFcn=NIVeriStand_MDL_functions('', 'IO_delete');  MoveFcn=set_param(gcb, 'Mask', 'on');
      mask Callback portnum: NIVeriStand_MDL_functions('', 'IO_setportnum');
      mask TypeOptions dtype: auto | double | single | int8 | uint8 | int16 | uint16 | int32 | uint32 | boolean
      mask Callback dtype: NIVeriStand_MDL_functions('', 'IO_booleansignal');
      mask TypeOptions stype: auto | real | complex
      mask Display:
      | patch([-x x], [-y y], [.90980 .81960 .32156]);
      | plot([xrad -x x xrad], [yrad -y y yrad]);
      | fprintf('NI Out%d', portnum);
  "psi_0 " : S-Function  Priority=4  FunctionName=NIVeriStandIO  Parameters=width dtype portnum stime stype btype  mask(NI VeriStand Outport){portnum=4, width=-1, stime=-1, dtype=auto, stype=auto, btype=0}
      mask prompts: portnum "Port number:"; width "Port dimensions (-1 for dynamically sized):"; stime "Sample time (-1 for inherited):"; dtype "Data type:"; stype "Signal type:"; btype "Block type:"
      mask help: Use this outport on any level of nested subsystems to allow NI VeriStand software to map signals to it.
      mask init:
      | NIVeriStandIO_init;
      settings: CopyFcn=NIVeriStand_MDL_functions('', 'IO_copy');  DeleteFcn=NIVeriStand_MDL_functions('', 'IO_delete');  MoveFcn=set_param(gcb, 'Mask', 'on');
      mask Callback portnum: NIVeriStand_MDL_functions('', 'IO_setportnum');
      mask TypeOptions dtype: auto | double | single | int8 | uint8 | int16 | uint16 | int32 | uint32 | boolean
      mask Callback dtype: NIVeriStand_MDL_functions('', 'IO_booleansignal');
      mask TypeOptions stype: auto | real | complex
      mask Display:
      | patch([-x x], [-y y], [.90980 .81960 .32156]);
      | plot([xrad -x x xrad], [yrad -y y yrad]);
      | fprintf('NI Out%d', portnum);
  x_0 : S-Function  Priority=5  FunctionName=NIVeriStandIO  Parameters=width dtype portnum stime stype btype  mask(NI VeriStand Outport){portnum=5, width=-1, stime=-1, dtype=auto, stype=auto, btype=0}
      mask prompts: portnum "Port number:"; width "Port dimensions (-1 for dynamically sized):"; stime "Sample time (-1 for inherited):"; dtype "Data type:"; stype "Signal type:"; btype "Block type:"
      mask help: Use this outport on any level of nested subsystems to allow NI VeriStand software to map signals to it.
      mask init:
      | NIVeriStandIO_init;
      settings: CopyFcn=NIVeriStand_MDL_functions('', 'IO_copy');  DeleteFcn=NIVeriStand_MDL_functions('', 'IO_delete');  MoveFcn=set_param(gcb, 'Mask', 'on');
      mask Callback portnum: NIVeriStand_MDL_functions('', 'IO_setportnum');
      mask TypeOptions dtype: auto | double | single | int8 | uint8 | int16 | uint16 | int32 | uint32 | boolean
      mask Callback dtype: NIVeriStand_MDL_functions('', 'IO_booleansignal');
      mask TypeOptions stype: auto | real | complex
      mask Display:
      | patch([-x x], [-y y], [.90980 .81960 .32156]);
      | plot([xrad -x x xrad], [yrad -y y yrad]);
      | fprintf('NI Out%d', portnum);
  y_0 : S-Function  Priority=6  FunctionName=NIVeriStandIO  Parameters=width dtype portnum stime stype btype  mask(NI VeriStand Outport){portnum=6, width=-1, stime=-1, dtype=auto, stype=auto, btype=0}
      mask prompts: portnum "Port number:"; width "Port dimensions (-1 for dynamically sized):"; stime "Sample time (-1 for inherited):"; dtype "Data type:"; stype "Signal type:"; btype "Block type:"
      mask help: Use this outport on any level of nested subsystems to allow NI VeriStand software to map signals to it.
      mask init:
      | NIVeriStandIO_init;
      settings: CopyFcn=NIVeriStand_MDL_functions('', 'IO_copy');  DeleteFcn=NIVeriStand_MDL_functions('', 'IO_delete');  MoveFcn=set_param(gcb, 'Mask', 'on');
      mask Callback portnum: NIVeriStand_MDL_functions('', 'IO_setportnum');
      mask TypeOptions dtype: auto | double | single | int8 | uint8 | int16 | uint16 | int32 | uint32 | boolean
      mask Callback dtype: NIVeriStand_MDL_functions('', 'IO_booleansignal');
      mask TypeOptions stype: auto | real | complex
      mask Display:
      | patch([-x x], [-y y], [.90980 .81960 .32156]);
      | plot([xrad -x x xrad], [yrad -y y yrad]);
      | fprintf('NI Out%d', portnum);
  wires:
  tau_d to model/1 -> Demux/1
  Demux/1 -> X_d/1
  Demux/2 -> Y_d/1
  Demux/3 -> N_d/1
  Constant2/1 -> "psi_0 "/1
  Constant1/1 -> y_0/1
  Constant/1 -> x_0/1
  integrator reset/1 -> integrator reset model/1

== system ctrl_student_HIL/Noise generator/Downsample	signal ==
  sampling frequency : Inport
  step size : Inport  Port=2
  MATLAB Function : MATLAB Function  TreatAsAtomicUnit=on
  counter : Memory
  trigger : Outport
  wires:
  sampling frequency/1 -> MATLAB Function/1(f)
  step size/1 -> MATLAB Function/2(h)
  counter/1 -> MATLAB Function/3(i)
  MATLAB Function/1(count) -> counter/1, trigger/1

== system ctrl_student_HIL/Noise generator/Sample & hold ==
  trigger : Inport
  input : Inport  Port=2
  Hold : Memory
  MATLAB Function1 : MATLAB Function  TreatAsAtomicUnit=on
  output : Outport
  wires:
  MATLAB Function1/1(output) -> output/1, Hold/1
  trigger/1 -> MATLAB Function1/1(counter)
  input/1 -> MATLAB Function1/2(input)
  Hold/1 -> MATLAB Function1/3(hold)

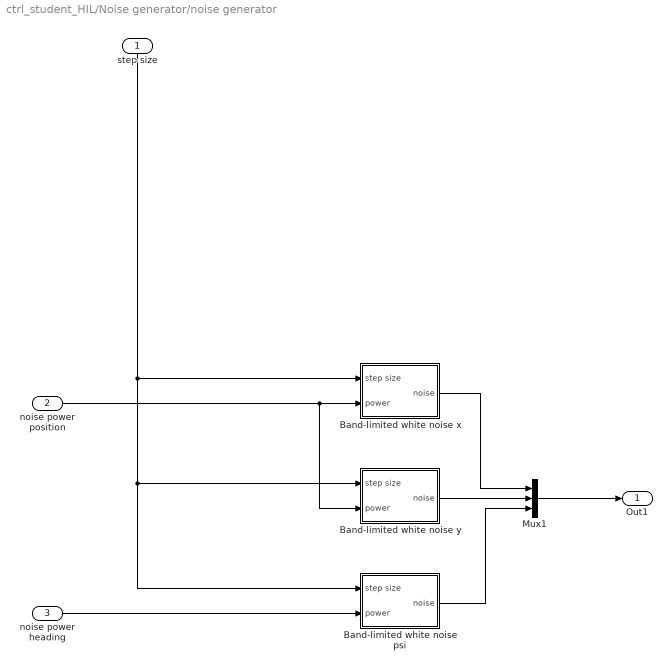
== system ctrl_student_HIL/Noise generator/noise generator ==
  step size : Inport
  noise power position : Inport  Port=2
  noise power heading : Inport  Port=3
  Band-limited white noise psi : Subsystem
  Band-limited white noise x : Subsystem
  Band-limited white noise y : Subsystem
  Mux1 : Mux  Inputs=3
  Out1 : Outport
  wires:
  Mux1/1 -> Out1/1
  step size/1 -> Band-limited white noise x/1(step size), Band-limited white noise psi/1(step size), Band-limited white noise y/1(step size)
  noise power position/1 -> Band-limited white noise y/2(power), Band-limited white noise x/2(power)
  Band-limited white noise x/1(noise) -> Mux1/1
  Band-limited white noise y/1(noise) -> Mux1/2
  Band-limited white noise psi/1(noise) -> Mux1/3
  noise power heading/1 -> Band-limited white noise psi/2(power)

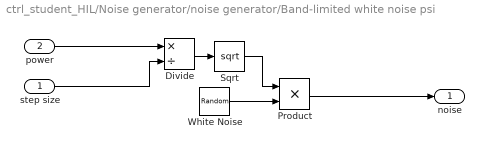
== system ctrl_student_HIL/Noise generator/noise generator/Band-limited white noise psi ==
  step size : Inport
  power : Inport  Port=2
  Divide : Product  Inputs=*/
  Product : Product
  Sqrt : Sqrt  SaturateOnIntegerOverflow=on
  White Noise : RandomNumber  DisableCoverage=on  Seed=9025
  noise : Outport
  wires:
  White Noise/1 -> Product/2
  Product/1 -> noise/1
  step size/1 -> Divide/2
  Divide/1 -> Sqrt/1
  Sqrt/1 -> Product/1
  power/1 -> Divide/1

== system ctrl_student_HIL/Noise generator/noise generator/Band-limited white noise x ==
  step size : Inport
  power : Inport  Port=2
  Divide : Product  Inputs=*/
  Product : Product
  Sqrt : Sqrt  SaturateOnIntegerOverflow=on
  White Noise : RandomNumber  DisableCoverage=on  Seed=9024
  noise : Outport
  wires:
  White Noise/1 -> Product/2
  Product/1 -> noise/1
  step size/1 -> Divide/2
  Divide/1 -> Sqrt/1
  Sqrt/1 -> Product/1
  power/1 -> Divide/1

== system ctrl_student_HIL/Noise generator/noise generator/Band-limited white noise y ==
  step size : Inport
  power : Inport  Port=2
  Divide : Product  Inputs=*/
  Product : Product
  Sqrt : Sqrt  SaturateOnIntegerOverflow=on
  White Noise : RandomNumber  DisableCoverage=on  Seed=123
  noise : Outport
  wires:
  White Noise/1 -> Product/2
  Product/1 -> noise/1
  step size/1 -> Divide/2
  Divide/1 -> Sqrt/1
  Sqrt/1 -> Product/1
  power/1 -> Divide/1
